simulink library "Contact_Forces_Lib"  (R2016a)
settings: Solver=ode45  StartTime=0.0  StopTime=10.0  RelTol=1e-3
undefined symbols (not defined in the file or in its folder): Extr_Data_Ring, radius_tube, X, Y, Z
undefined symbols (not defined in the file): b_contact, custom_param_1, custom_param_2, k_contact, l_cone, length_cylinder, length_tube, mu_kinetic, mu_static, pen_exponent, pen_full_damp_F, rad_s_cone, radius_cylinder, v_thr
libraries: nesl_utility x200, sm_lib x115, Contact_Forces_Lib x72, simulink x20, fl_lib x1
(part 10 of 12)

== system Contact_Forces_Lib/2D/Circle to Finite Line Force Enabled/Forces/Resolve Forces/Friction ==
  Unit Vector : Inport
  Fn : Inport  Port=2
  X Sep : Inport  Port=3
  vLin : Inport  Port=4
  wz : Inport  Port=5
  Components : Gain  Gain=[1 -1]
  Demux : Demux  Outputs=2
  Friction Law : Contact_Forces_Lib/Friction Law  OverrideUsingVariant=None
  Line Ref h : Gain  Gain=line_depth
  Product1 : Product
  Product2 : Product
  Product3 : Product
  Radius : Gain  Gain=-circle_rad
  Sign : Signum
  Sum : Sum  Inputs=-+
  VCirPt : Subsystem
  FxCir : Outport
  FyCir : Outport  Port=2
  FyLin : Outport  Port=3
  TzLin : Outport  Port=4
  TzCir : Outport  Port=5
  Ff : Outport  Port=6
  wires:
  Product3/1 -> Product2/1
  Components/1 -> Product3/1
  Product1/1 -> FyLin/1
  Friction Law/1 -> Line Ref h/1, Product2/2, Ff/1, Radius/1, Product1/1  "Ff"
  Demux/1 -> FyCir/1  "FyCir"
  vLin/1 -> Sum/1
  VCirPt/1(vCir) -> Sum/2
  Demux/2 -> FxCir/1  "FxCir"
  wz/1 -> VCirPt/1(wz)
  Unit Vector/1 -> Components/1
  Sum/1 -> Friction Law/2
  Fn/1 -> Friction Law/1
  Line Ref h/1 -> TzLin/1
  Radius/1 -> TzCir/1
  Product2/1 -> Demux/1
  X Sep/1 -> Sign/1, VCirPt/2(X sep)
  Sign/1 -> Product1/2, Product3/2

== system Contact_Forces_Lib/2D/Circle to Ring Force/Forces/Ff/Calculate vRel at CP  ==
  InOut : Inport
  rad : Inport  Port=2
  Pen : Inport  Port=3
  vazm : Inport  Port=4
  wzf : Inport  Port=5
  Follower Radius : Constant  Value=radius_circle
  Midpt Pen : Gain  Gain=0.5
  Product1 : Product
  Product2 : Product
  Product3 : Product
  Sum{,1..2,4} (4 alike) : Sum  Inputs=+-
  vRelCP : Outport
  rCirFtoCP : Outport  Port=2
  rRinBtoCP : Outport  Port=3
  wires:
  InOut/1 -> Product1/2  "InOut"
  Sum2/1 -> vRelCP/1
  Pen/1 -> Midpt Pen/1
  Sum/1 -> rRinBtoCP/1, Product2/2  "rRinBtoCP"
  rad/1 -> Sum/1
  Product2/1 -> Sum2/1  "vRelTra"
  Product3/1 -> Sum2/2  "vRelRot"
  Follower Radius/1 -> Sum1/1
  wzf/1 -> Sum4/1
  vazm/1 -> Product2/1, Sum4/2
  Midpt Pen/1 -> Sum1/2
  Sum4/1 -> Product3/1
  Product1/1 -> Sum/2, Product3/2  "rCirFtoCP sign"
  Sum1/1 -> rCirFtoCP/1, Product1/1  "rCirFtoCP"

== system Contact_Forces_Lib/2D/Circle to Ring Force/Forces/Ff/Resolve Ff ==
  note: Resolve Friction Force in
      | Circle B reference frame
      | Sign of Fn indicates
      | inside or outside ring.
  note: Resolve Friction Force in
      | Circle F reference frame
  Fn : Inport
  Ff : Inport  Port=2
  R : Inport  Port=3
  azm : Inport  Port=4
  rCirFtoCP : Inport  Port=5
  rRinBtoCP : Inport  Port=6
  Ff in CirB : Subsystem
  Ff in CirF : Subsystem
  Product : Product
  Sign : Signum  ZeroCross=off
  Tz : Subsystem
  FxCirF : Outport
  FyCirF : Outport  Port=2
  TzCirF : Outport  Port=3
  FxRinB : Outport  Port=4
  FyRinB : Outport  Port=5
  TzRinB : Outport  Port=6
  wires:
  Product/1 -> Ff in CirB/1(Ff)
  Sign/1 -> Product/2
  Fn/1 -> Sign/1
  Ff in CirF/1(FyCirF) -> FyCirF/1
  Ff in CirB/1(FxRinB) -> FxRinB/1, Ff in CirF/2(FxRinB)
  Ff in CirB/2(FyRinB) -> FyRinB/1, Ff in CirF/3(FyRinB)
  Ff in CirF/2(FxCirF) -> FxCirF/1
  Ff/1 -> Product/1, Tz/3(Ff)
  Tz/1(TzRinB) -> TzRinB/1
  Tz/2(TzCirF) -> TzCirF/1
  azm/1 -> Ff in CirB/2(azm)
  R/1 -> Ff in CirF/1(R)
  rCirFtoCP/1 -> Tz/1(rCirFtoCP)
  rRinBtoCP/1 -> Tz/2(rRinBtoCP)

== system Contact_Forces_Lib/2D/Circle to Ring Force/Forces/Fn/Fn in CirB ==
  Fn : Inport
  azm : Inport  Port=2
  Divide1 : Product  Inputs=**
  Divide2 : Product  Inputs=**
  Gain2 : Gain  Gain=-1
  cos : Trigonometry  Operator=cos
  deg2rad : Gain  Gain=pi/180
  sin : Trigonometry
  FxCirB : Outport
  FyCirB : Outport  Port=2
  wires:
  Gain2/1 -> Divide1/1, Divide2/1
  deg2rad/1 -> cos/1, sin/1
  sin/1 -> Divide2/2
  cos/1 -> Divide1/2
  Divide1/1 -> FxCirB/1
  Divide2/1 -> FyCirB/1
  Fn/1 -> Gain2/1
  azm/1 -> deg2rad/1

== system Contact_Forces_Lib/2D/Circle to Ring Force/Forces/Fn/Fn in CirF ==
  R : Inport
  FxCirB : Inport  Port=2
  FyCirB : Inport  Port=3
  Demux : Demux  Outputs=2
  Divide3 : Product  Inputs=**  Multiplication=Matrix(*)
  Gain : Gain  Gain=-1
  Mux1 : Mux  Inputs=2
  FyCirF : Outport
  FxCirF : Outport  Port=2
  wires:
  Demux/2 -> FxCirF/1
  Demux/1 -> FyCirF/1
  Gain/1 -> Demux/1
  Mux1/1 -> Divide3/2
  Divide3/1 -> Gain/1
  R/1 -> Divide3/1
  FyCirB/1 -> Mux1/1
  FxCirB/1 -> Mux1/2

== system Contact_Forces_Lib/2D/Composite Forces/Box to Belt Force/Belt Ends/Sensing C5 ==
  S : Inport
  Bus Selector : BusSelector  OutputSignals=Normal Force
  Fn : Outport
  wires:
  S/1 -> Bus Selector/1
  Bus Selector/1 -> Fn/1  "<Normal Force>"

== system Contact_Forces_Lib/2D/Composite Forces/Box to Belt Force/Belt Ends/Sensing C6 ==
  S : Inport
  Bus Selector : BusSelector  OutputSignals=Normal Force
  Fn : Outport
  wires:
  Bus Selector/1 -> Fn/1  "<Normal Force>"
  S/1 -> Bus Selector/1

== system Contact_Forces_Lib/2D/Composite Forces/Box to Belt Force/Belt Ends/Sensing C7 ==
  S : Inport
  Bus Selector : BusSelector  OutputSignals=Normal Force
  Fn : Outport
  wires:
  Bus Selector/1 -> Fn/1  "<Normal Force>"
  S/1 -> Bus Selector/1

== system Contact_Forces_Lib/2D/Composite Forces/Box to Belt Force/Belt Ends/Sensing C8 ==
  S : Inport
  Bus Selector : BusSelector  OutputSignals=Normal Force
  Fn : Outport
  wires:
  S/1 -> Bus Selector/1
  Bus Selector/1 -> Fn/1  "<Normal Force>"

== system Contact_Forces_Lib/2D/Composite Forces/Box to Belt Force/Belt Faces/Sensing C1 ==
  S : Inport
  Bus Selector : BusSelector  OutputSignals=Normal Force
  Fn : Outport
  wires:
  Bus Selector/1 -> Fn/1  "<Normal Force>"
  S/1 -> Bus Selector/1

== system Contact_Forces_Lib/2D/Composite Forces/Box to Belt Force/Belt Faces/Sensing C2 ==
  S : Inport
  Bus Selector : BusSelector  OutputSignals=Normal Force
  Fn : Outport
  wires:
  S/1 -> Bus Selector/1
  Bus Selector/1 -> Fn/1  "<Normal Force>"

== system Contact_Forces_Lib/2D/Composite Forces/Box to Belt Force/Belt Faces/Sensing C3 ==
  S : Inport
  Bus Selector : BusSelector  OutputSignals=Normal Force
  Fn : Outport
  wires:
  S/1 -> Bus Selector/1
  Bus Selector/1 -> Fn/1  "<Normal Force>"

== system Contact_Forces_Lib/2D/Composite Forces/Box to Belt Force/Belt Faces/Sensing C4 ==
  S : Inport
  Bus Selector : BusSelector  OutputSignals=Normal Force
  Fn : Outport
  wires:
  Bus Selector/1 -> Fn/1  "<Normal Force>"
  S/1 -> Bus Selector/1

== system Contact_Forces_Lib/2D/Composite Forces/Box to Box Force/BoxB Corners/Forces ==
  1AC : Inport
  1BD : Inport  Port=2
  2AC : Inport  Port=3
  2BD : Inport  Port=4
  3AC : Inport  Port=5
  3BD : Inport  Port=6
  4AC : Inport  Port=7
  4BD : Inport  Port=8
  Bus Creator : BusCreator  Inputs=8
  Bus Selector{1..8} (8 alike) : BusSelector  OutputSignals=FLin.Fx  OutputAsBus=on
  tag scope: FrcBC=scoped
  wires:
  Bus Creator/1 -> [FrcBC]
  Bus Selector7/1 -> Bus Creator/8  "BC4BD"
  4BD/1 -> Bus Selector7/1
  Bus Selector8/1 -> Bus Creator/7  "BC4AC"
  4AC/1 -> Bus Selector8/1
  Bus Selector5/1 -> Bus Creator/6  "BC3BD"
  3BD/1 -> Bus Selector5/1
  Bus Selector6/1 -> Bus Creator/5  "BC3AC"
  3AC/1 -> Bus Selector6/1
  Bus Selector3/1 -> Bus Creator/4  "BC2BD"
  2BD/1 -> Bus Selector3/1
  Bus Selector4/1 -> Bus Creator/3  "BC2AC"
  2AC/1 -> Bus Selector4/1
  Bus Selector1/1 -> Bus Creator/2  "BC1BD"
  1BD/1 -> Bus Selector1/1
  Bus Selector2/1 -> Bus Creator/1  "BC1AC"
  1AC/1 -> Bus Selector2/1

== system Contact_Forces_Lib/2D/Composite Forces/Box to Box Force/BoxF Corners/Forces ==
  1AC : Inport
  1BD : Inport  Port=2
  2AC : Inport  Port=3
  2BD : Inport  Port=4
  3AC : Inport  Port=5
  3BD : Inport  Port=6
  4AC : Inport  Port=7
  4BD : Inport  Port=8
  Bus Creator : BusCreator  Inputs=8
  Bus Selector{1..8} (8 alike) : BusSelector  OutputSignals=FLin.Fx  OutputAsBus=on
  tag scope: FrcFC=scoped
  wires:
  Bus Creator/1 -> [FrcFC]
  Bus Selector7/1 -> Bus Creator/8  "FC4BD"
  4BD/1 -> Bus Selector7/1
  Bus Selector8/1 -> Bus Creator/7  "FC4AC"
  4AC/1 -> Bus Selector8/1
  Bus Selector5/1 -> Bus Creator/6  "FC3BD"
  3BD/1 -> Bus Selector5/1
  Bus Selector6/1 -> Bus Creator/5  "FC3AC"
  3AC/1 -> Bus Selector6/1
  Bus Selector3/1 -> Bus Creator/4  "FC2BD"
  2BD/1 -> Bus Selector3/1
  Bus Selector4/1 -> Bus Creator/3  "FC2AC"
  2AC/1 -> Bus Selector4/1
  Bus Selector1/1 -> Bus Creator/2  "FC1BD"
  1BD/1 -> Bus Selector1/1
  Bus Selector2/1 -> Bus Creator/1  "FC1AC"
  1AC/1 -> Bus Selector2/1

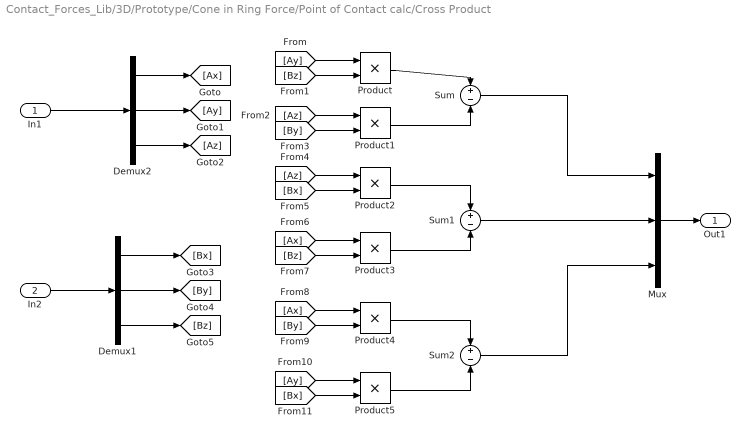
== system Contact_Forces_Lib/3D/Prototype/Cone in Ring Force/Point of Contact calc/Cross Product ==
  In1 : Inport
  In2 : Inport  Port=2
  Demux1 : Demux  Outputs=3
  Demux2 : Demux  Outputs=3
  Mux : Mux  Inputs=3
  Product{,1..5} (6 alike) : Product
  Sum : Sum  Inputs=+|-
  Sum1 : Sum  Inputs=+|-
  Sum2 : Sum  Inputs=+|-
  Out1 : Outport
  wires:
  [Bx] -> Product5/2
  [Ay] -> Product5/1
  [By] -> Product4/2
  [Ax] -> Product4/1
  [Bz] -> Product3/2
  [Ax] -> Product3/1
  [Bx] -> Product2/2
  [Az] -> Product2/1
  [By] -> Product1/2
  [Az] -> Product1/1
  [Bz] -> Product/2
  [Ay] -> Product/1
  Demux1/3 -> [Bz]
  Demux1/2 -> [By]
  Demux1/1 -> [Bx]
  Demux2/3 -> [Az]
  Demux2/2 -> [Ay]
  Demux2/1 -> [Ax]
  In1/1 -> Demux2/1
  Sum2/1 -> Mux/3
  Sum/1 -> Mux/1
  Sum1/1 -> Mux/2
  Product5/1 -> Sum2/2
  Product4/1 -> Sum2/1
  Product3/1 -> Sum1/2
  Product2/1 -> Sum1/1
  Product/1 -> Sum/1
  Product1/1 -> Sum/2
  Mux/1 -> Out1/1
  In2/1 -> Demux1/1

== system Contact_Forces_Lib/3D/Prototype/Cone in Ring Force/Point of Contact calc/Force Calc ==
  x : Inport
  y : Inport  Port=2
  r : Inport  Port=3
  z : Inport  Port=4
  th : Inport  Port=5
  Computing Force from nonzero penetration points : Subsystem  Commented=on
  Constant2 : Constant  Value=r_tube
  Dead Zone : DeadZone  LowerValue=-inf  UpperValue=0  ZeroCross=off  SaturateOnIntegerOverflow=on
  MAX_ML : Subsystem  Commented=on
  MAX_SL : Subsystem
  Math Function : Math  Operator=square  SaturateOnIntegerOverflow=on
  Math Function1 : Math  Operator=square  SaturateOnIntegerOverflow=on
  Reciprocal Sqrt : Sqrt  SaturateOnIntegerOverflow=on
  Sum : Sum  Inputs=|++
  Sum1 : Sum  Inputs=|+-
  Fx : Outport
  Fy : Outport  Port=2
  Fz : Outport  Port=3
  pc : Outport  Port=4
  wires:
  x/1 -> MAX_SL/2(X), Math Function/1
  Sum/1 -> Reciprocal Sqrt/1
  Reciprocal Sqrt/1 -> Sum1/1
  Constant2/1 -> Sum1/2
  Sum1/1 -> Dead Zone/1
  Math Function1/1 -> Sum/1
  Math Function/1 -> Sum/2
  y/1 -> Math Function1/1, MAX_SL/1(Y)
  MAX_SL/1(Fx) -> Fx/1
  MAX_SL/2(Fy) -> Fy/1
  Dead Zone/1 -> MAX_SL/3(Pen)
  MAX_SL/3(Fz) -> Fz/1
  MAX_SL/4(pc) -> pc/1
  r/1 -> MAX_SL/4(r)
  th/1 -> MAX_SL/5(th)
  z/1 -> MAX_SL/6(z)

== system Contact_Forces_Lib/3D/Prototype/Cone in Ring Force/Point of Contact calc/r calc ==
  note: r(z) = (z+l_cyl/2)(rl-rs)/lc +rl
  z : Inport
  Constant4 : Constant  Value=(rl + (l_cyl*(rl - rs))/(2*lc))
  Gain1 : Gain  Gain=(rl - rs)/lc
  Sum1 : Sum  Inputs=|++
  r : Outport
  wires:
  Constant4/1 -> Sum1/2
  Gain1/1 -> Sum1/1
  z/1 -> Gain1/1
  Sum1/1 -> r/1

== system Contact_Forces_Lib/3D/Prototype/Cone in Ring Force/Point of Contact calc/x calc ==
  r11 : Inport
  r12 : Inport  Port=2
  r13 : Inport  Port=3
  xc : Inport  Port=4
  th : Inport  Port=5
  z : Inport  Port=6
  r : Inport  Port=7
  Product{,1..4} (5 alike) : Product
  Sum : Sum  Inputs=|++++
  Trigonometric Function : Trigonometry  Operator=cos
  Trigonometric Function1 : Trigonometry
  x : Outport
  wires:
  th/1 -> Trigonometric Function1/1, Trigonometric Function/1
  Sum/1 -> x/1
  Product/1 -> Product3/1
  Product4/1 -> Sum/3
  Trigonometric Function/1 -> Product/2
  Trigonometric Function1/1 -> Product1/2
  Product3/1 -> Sum/2
  Product1/1 -> Product4/2
  r11/1 -> Product/1
  r12/1 -> Product1/1
  xc/1 -> Sum/1
  r13/1 -> Product2/1
  z/1 -> Product2/2
  Product2/1 -> Sum/4
  r/1 -> Product3/2, Product4/1

== system Contact_Forces_Lib/3D/Prototype/Cone in Ring Force/Point of Contact calc/y calc ==
  r21 : Inport
  r22 : Inport  Port=2
  r23 : Inport  Port=3
  yc : Inport  Port=4
  th : Inport  Port=5
  z : Inport  Port=6
  r : Inport  Port=7
  Product{,1..4} (5 alike) : Product
  Sum : Sum  Inputs=|++++
  Trigonometric Function : Trigonometry  Operator=cos
  Trigonometric Function1 : Trigonometry
  y : Outport
  wires:
  Product2/1 -> Sum/4
  z/1 -> Product2/2
  r23/1 -> Product2/1
  yc/1 -> Sum/1
  r22/1 -> Product1/1
  r21/1 -> Product/1
  Product1/1 -> Product4/2
  Product3/1 -> Sum/2
  Trigonometric Function1/1 -> Product1/2
  Trigonometric Function/1 -> Product/2
  Product4/1 -> Sum/3
  Product/1 -> Product3/1
  Sum/1 -> y/1
  th/1 -> Trigonometric Function1/1, Trigonometric Function/1
  r/1 -> Product3/2, Product4/1

== system Contact_Forces_Lib/3D/Prototype/Cone in Ring Force/Point of Contact calc/z calc ==
  note: num = -(Zc - L/2 + r31*cos(th)*(rl + (Lcyl*(rl - rs))/(2*lc)) + r32*sin(th)*(rl + (Lcyl*(rl - rs))/(2*lc)))
      | den = (r33 + (r31*cos(th)*(rl - rs))/lc + (r32*sin(th)*(rl - rs))/lc)
  r31 : Inport
  r32 : Inport  Port=2
  r33 : Inport  Port=3
  zc : Inport  Port=4
  th : Inport  Port=5
  Constant : Constant  Value=(rl + (l_cyl*(rl - rs))/(2*lc))
  Constant1 : Constant  Value=l_tube/2
  Constant2 : Constant  Value=(rl - rs)/lc
  Divide : Product  Inputs=*/
  Gain : Gain  Gain=-1
  Product{,1..5} (6 alike) : Product
  Sum : Sum  Inputs=+-++
  Sum1 : Sum  Inputs=+++
  Trigonometric Function : Trigonometry  Operator=cos
  Trigonometric Function1 : Trigonometry
  z : Outport
  wires:
  Divide/1 -> z/1
  th/1 -> Trigonometric Function1/1, Trigonometric Function/1
  Trigonometric Function/1 -> Product/2
  r31/1 -> Product/1
  Trigonometric Function1/1 -> Product1/2
  r32/1 -> Product1/1
  zc/1 -> Sum/1
  Constant1/1 -> Sum/2
  Product2/1 -> Sum/3
  Product3/1 -> Sum/4
  Product/1 -> Product4/1, Product2/1
  Product1/1 -> Product3/1, Product5/1
  Constant/1 -> Product3/2, Product2/2
  Sum/1 -> Gain/1
  Product5/1 -> Sum1/3
  Product4/1 -> Sum1/2
  r33/1 -> Sum1/1
  Constant2/1 -> Product4/2, Product5/2
  Sum1/1 -> Divide/2
  Gain/1 -> Divide/1

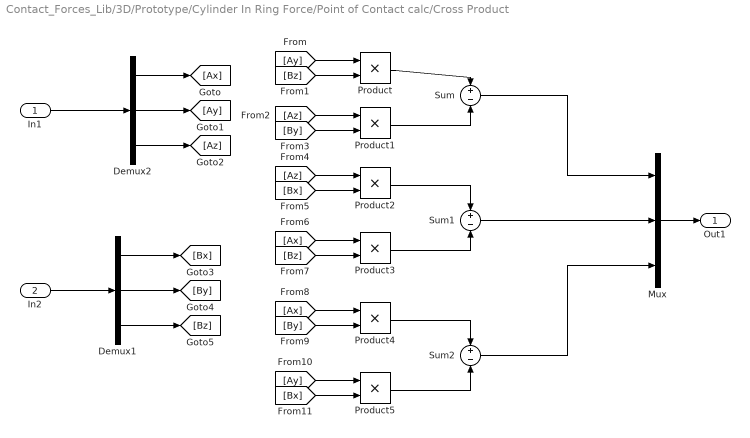
== system Contact_Forces_Lib/3D/Prototype/Cylinder In Ring Force/Point of Contact calc/Cross Product ==
  In1 : Inport
  In2 : Inport  Port=2
  Demux1 : Demux  Outputs=3
  Demux2 : Demux  Outputs=3
  Mux : Mux  Inputs=3
  Product{,1..5} (6 alike) : Product
  Sum : Sum  Inputs=+|-
  Sum1 : Sum  Inputs=+|-
  Sum2 : Sum  Inputs=+|-
  Out1 : Outport
  wires:
  [Bx] -> Product5/2
  [Ay] -> Product5/1
  [By] -> Product4/2
  [Ax] -> Product4/1
  [Bz] -> Product3/2
  [Ax] -> Product3/1
  [Bx] -> Product2/2
  [Az] -> Product2/1
  [By] -> Product1/2
  [Az] -> Product1/1
  [Bz] -> Product/2
  [Ay] -> Product/1
  Demux1/3 -> [Bz]
  Demux1/2 -> [By]
  Demux1/1 -> [Bx]
  Demux2/3 -> [Az]
  Demux2/2 -> [Ay]
  Demux2/1 -> [Ax]
  In1/1 -> Demux2/1
  Sum2/1 -> Mux/3
  Sum/1 -> Mux/1
  Sum1/1 -> Mux/2
  Product5/1 -> Sum2/2
  Product4/1 -> Sum2/1
  Product3/1 -> Sum1/2
  Product2/1 -> Sum1/1
  Product/1 -> Sum/1
  Product1/1 -> Sum/2
  Mux/1 -> Out1/1
  In2/1 -> Demux1/1

== system Contact_Forces_Lib/3D/Prototype/Cylinder In Ring Force/Point of Contact calc/Force Calc ==
  x : Inport
  y : Inport  Port=2
  v : Inport  Port=3
  z : Inport  Port=4
  th : Inport  Port=5
  Computing Force from nonzero penetration points : Subsystem  Commented=on
  Constant2 : Constant  Value=r_tube
  Dead Zone : DeadZone  LowerValue=-inf  UpperValue=0  ZeroCross=off  SaturateOnIntegerOverflow=on
  MAX_ML : Subsystem  Commented=on
  MAX_SL : Subsystem
  Math Function : Math  Operator=square  SaturateOnIntegerOverflow=on
  Math Function1 : Math  Operator=square  SaturateOnIntegerOverflow=on
  Reciprocal Sqrt : Sqrt  SaturateOnIntegerOverflow=on
  Sum : Sum  Inputs=|++
  Sum1 : Sum  Inputs=|+-
  Fx : Outport
  Fy : Outport  Port=2
  Fz : Outport  Port=3
  pc : Outport  Port=4
  maxpen : Outport  Port=5
  wires:
  y/1 -> MAX_SL/1(Y), Math Function1/1
  x/1 -> MAX_SL/2(X), Math Function/1
  Sum/1 -> Reciprocal Sqrt/1
  Reciprocal Sqrt/1 -> Sum1/1
  Constant2/1 -> Sum1/2
  Sum1/1 -> Dead Zone/1
  MAX_SL/1(Fx) -> Fx/1
  MAX_SL/2(Fy) -> Fy/1
  Dead Zone/1 -> MAX_SL/3(Pen)
  Math Function1/1 -> Sum/1
  Math Function/1 -> Sum/2
  v/1 -> MAX_SL/4(v)
  th/1 -> MAX_SL/5(th)
  z/1 -> MAX_SL/6(z)
  MAX_SL/4(pc) -> pc/1
  MAX_SL/3(Fz) -> Fz/1
  MAX_SL/5(maxpen) -> maxpen/1

== system Contact_Forces_Lib/3D/Prototype/Cylinder In Ring Force/Point of Contact calc/x calc ==
  note: Xb = r11*r*cos(th) + r12*r*sin(th) +r13*z + Xc;
  note: Find x coordinate in tube frame for cylinder point that is in the plane of the end of the tube
  r11 : Inport
  r12 : Inport  Port=2
  r13 : Inport  Port=3
  xc : Inport  Port=4
  th : Inport  Port=5
  z : Inport  Port=6
  Gain : Gain  Gain=r_cyl
  Gain1 : Gain  Gain=r_cyl
  Product : Product
  Product1 : Product
  Product2 : Product
  Sum : Sum  Inputs=|++++
  Trigonometric Function : Trigonometry  Operator=cos
  Trigonometric Function1 : Trigonometry
  x : Outport
  wires:
  th/1 -> Trigonometric Function/1, Trigonometric Function1/1
  Sum/1 -> x/1
  Product/1 -> Gain/1
  Gain1/1 -> Sum/3
  Trigonometric Function/1 -> Product/2
  Trigonometric Function1/1 -> Product1/2
  Gain/1 -> Sum/2
  Product1/1 -> Gain1/1
  r11/1 -> Product/1
  r12/1 -> Product1/1
  xc/1 -> Sum/1
  r13/1 -> Product2/1
  z/1 -> Product2/2
  Product2/1 -> Sum/4

== system Contact_Forces_Lib/3D/Prototype/Cylinder In Ring Force/Point of Contact calc/y calc ==
  note: Yb = r21*r*cos(th) + r22*r*sin(th) +r23*z + Yc;
  note: Find y coordinate in tube frame for cylinder point that is in the plane of the end of the tube
  r21 : Inport
  r22 : Inport  Port=2
  r23 : Inport  Port=3
  yc : Inport  Port=4
  th : Inport  Port=5
  z : Inport  Port=6
  Gain : Gain  Gain=r_cyl
  Gain1 : Gain  Gain=r_cyl
  Product : Product
  Product1 : Product
  Product2 : Product
  Sum : Sum  Inputs=|++++
  Trigonometric Function : Trigonometry  Operator=cos
  Trigonometric Function1 : Trigonometry
  y : Outport
  wires:
  Product2/1 -> Sum/4
  z/1 -> Product2/2
  r23/1 -> Product2/1
  yc/1 -> Sum/1
  r22/1 -> Product1/1
  r21/1 -> Product/1
  Product1/1 -> Gain1/1
  Gain/1 -> Sum/2
  Trigonometric Function1/1 -> Product1/2
  Trigonometric Function/1 -> Product/2
  Gain1/1 -> Sum/3
  Product/1 -> Gain/1
  Sum/1 -> y/1
  th/1 -> Trigonometric Function1/1, Trigonometric Function/1

== system Contact_Forces_Lib/3D/Prototype/Cylinder In Ring Force/Point of Contact calc/z calc ==
  note: Find z coordinate in cylinder frame for cylinder point that is in the plane of the end of the tube
  note: z = (L/2 - r31*r*cos(th) - r32*r*sin(th) - Zc)/r33;
  r31 : Inport
  r32 : Inport  Port=2
  r33 : Inport  Port=3
  zc : Inport  Port=4
  th : Inport  Port=5
  Constant : Constant  Value=l_tube/2
  Divide : Product  Inputs=*/
  Gain : Gain  Gain=r_cyl
  Gain1 : Gain  Gain=r_cyl
  Product : Product
  Product1 : Product
  Sum : Sum  Inputs=|---+
  Trigonometric Function : Trigonometry  Operator=cos
  Trigonometric Function1 : Trigonometry
  z : Outport
  wires:
  r32/1 -> Product1/1
  r31/1 -> Product/1
  Product1/1 -> Gain1/1
  Gain/1 -> Sum/2
  Trigonometric Function1/1 -> Product1/2
  Trigonometric Function/1 -> Product/2
  Gain1/1 -> Sum/3
  Product/1 -> Gain/1
  r33/1 -> Divide/2
  Constant/1 -> Sum/4
  Sum/1 -> Divide/1
  Divide/1 -> z/1
  zc/1 -> Sum/1
  th/1 -> Trigonometric Function1/1, Trigonometric Function/1

== system Contact_Forces_Lib/3D/Sphere in Sphere Force/Ff/Check w or v non zero/Else ==
  Action Port : ActionPort
  vabs_zero : Constant  Value=0  SampleTime=0
  vuvect_zero : Constant  Value=[0 0 0]  SampleTime=0
  vabs : Outport  InitialOutput=0
  vuvect : Outport  Port=2  InitialOutput=0
  wires:
  vabs_zero/1 -> vabs/1
  vuvect_zero/1 -> vuvect/1

== system Contact_Forces_Lib/3D/Sphere in Sphere Force/Ff/Check w or v non zero/mag v ==
  vect : Inport
  Add2 : Sum  Inputs=+++
  Demux : Demux  Outputs=3
  Math Function : Math  Operator=square  SaturateOnIntegerOverflow=on
  Math Function1 : Math  Operator=square  SaturateOnIntegerOverflow=on
  Math Function2 : Math  Operator=square  SaturateOnIntegerOverflow=on
  Sqrt : Sqrt  SaturateOnIntegerOverflow=on
  mag : Outport
  wires:
  Math Function2/1 -> Add2/3
  Demux/3 -> Math Function2/1
  Sqrt/1 -> mag/1
  Math Function1/1 -> Add2/2
  Math Function/1 -> Add2/1
  Add2/1 -> Sqrt/1
  vect/1 -> Demux/1
  Demux/1 -> Math Function/1
  Demux/2 -> Math Function1/1

== system Contact_Forces_Lib/3D/Sphere in Sphere Force/Ff/Check w or v non zero/mag w ==
  vect : Inport
  Add : Sum  Inputs=+++
  Demux : Demux  Outputs=3
  Math Function : Math  Operator=square  SaturateOnIntegerOverflow=on
  Math Function1 : Math  Operator=square  SaturateOnIntegerOverflow=on
  Math Function2 : Math  Operator=square  SaturateOnIntegerOverflow=on
  Sqrt : Sqrt  SaturateOnIntegerOverflow=on
  mag : Outport
  wires:
  Demux/2 -> Math Function1/1
  Demux/1 -> Math Function/1
  vect/1 -> Demux/1
  Add/1 -> Sqrt/1
  Math Function/1 -> Add/1
  Math Function1/1 -> Add/2
  Sqrt/1 -> mag/1
  Demux/3 -> Math Function2/1
  Math Function2/1 -> Add/3

== system Contact_Forces_Lib/3D/Sphere in Sphere Force/Ff/SlipVel/If Action Subsystem ==
  In1 : Inport
  In2 : Inport  Port=2
  Action Port : ActionPort
  Divide : Product  Inputs=/*
  Out1 : Outport
  wires:
  Divide/1 -> Out1/1
  In2/1 -> Divide/2
  In1/1 -> Divide/1

== system Contact_Forces_Lib/3D/Sphere in Sphere Force/Ff/SlipVel/mag ==
  vect : Inport
  Add2 : Sum  Inputs=+++
  Demux : Demux  Outputs=3
  Math Function : Math  Operator=square  SaturateOnIntegerOverflow=on
  Math Function1 : Math  Operator=square  SaturateOnIntegerOverflow=on
  Math Function2 : Math  Operator=square  SaturateOnIntegerOverflow=on
  Sqrt : Sqrt  SaturateOnIntegerOverflow=on
  mag : Outport
  wires:
  Math Function2/1 -> Add2/3
  Demux/3 -> Math Function2/1
  Sqrt/1 -> mag/1
  Math Function1/1 -> Add2/2
  Math Function/1 -> Add2/1
  Add2/1 -> Sqrt/1
  vect/1 -> Demux/1
  Demux/1 -> Math Function/1
  Demux/2 -> Math Function1/1

== system Contact_Forces_Lib/3D/Sphere to Cone Force/Forces/Ff/Relative vel at CP ==
  note: Calculate relative velocity at contact point between sphere and tube. Two components: about ring and along tube axis. Use magnitude to calculate friction force, atan2 retains relative magnitude and direction between the components.
  InOut : Inport
  rad : Inport  Port=2
  vrad : Inport  Port=3
  Pen : Inport  Port=4
  vazm : Inport  Port=5
  vazmx : Inport  Port=6
  vazmy : Inport  Port=7
  wzf : Inport  Port=8
  vzf : Inport  Port=9
  wxf : Inport  Port=10
  wyf : Inport  Port=11
  azm : Inport  Port=12
  Calculate vRelFace : Subsystem
  Calculate vRelRing : Subsystem
  Follower Radius : Constant  Value=radius_sphere
  Math Function : Math  Operator=square  SaturateOnIntegerOverflow=on
  Math Function1 : Math  Operator=square  SaturateOnIntegerOverflow=on
  Midpt Pen : Gain  Gain=0.5
  Product1 : Product
  Sqrt : Sqrt  SaturateOnIntegerOverflow=on
  Sum1 : Sum  Inputs=+-
  Sum3 : Sum  Inputs=|++
  Trigonometric Function : Trigonometry  Operator=atan2
  vRelAbs : Outport
  rSphtoCP : Outport  Port=2
  rConAxtoCP : Outport  Port=3
  alpha : Outport  Port=4
  wires:
  vrad/1 -> Calculate vRelFace/6(vrad)
  vazmy/1 -> Calculate vRelRing/6(vazmy)
  vazmx/1 -> Calculate vRelRing/5(vazmx)
  Product1/1 -> Calculate vRelRing/1(rSphtoCP sign), Calculate vRelFace/1(rSphtoCP sign)
  Sum1/1 -> Product1/1, rSphtoCP/1  "rSphtoCP"
  InOut/1 -> Product1/2  "InOut"
  Trigonometric Function/1 -> alpha/1  "alpha"
  Sqrt/1 -> vRelAbs/1
  Sum3/1 -> Sqrt/1
  Math Function/1 -> Sum3/1
  Math Function1/1 -> Sum3/2
  Follower Radius/1 -> Sum1/1
  Pen/1 -> Midpt Pen/1
  Midpt Pen/1 -> Sum1/2
  Calculate vRelFace/1(vRelFace) -> Math Function1/1, Trigonometric Function/1  "vRelFace"
  wxf/1 -> Calculate vRelFace/3(wxf), Calculate vRelRing/8(wxf)
  vzf/1 -> Calculate vRelFace/5(vzf)
  azm/1 -> Calculate vRelFace/2(azm), Calculate vRelRing/7(azm)
  wyf/1 -> Calculate vRelRing/9(wyf), Calculate vRelFace/4(wyf)
  Calculate vRelRing/2(vRelRing) -> Math Function/1, Trigonometric Function/2  "vRelRing"
  rad/1 -> Calculate vRelRing/2(rad)
  vazm/1 -> Calculate vRelRing/3(vazm)
  wzf/1 -> Calculate vRelRing/4(wzf)
  Calculate vRelRing/1(rConAxtoCP) -> rConAxtoCP/1

== system Contact_Forces_Lib/3D/Sphere to Cone Force/Forces/Ff/Resolve Ff ==
  note: Resolve Friction Force in
      | Sphere F reference frame
  note: Resolve Friction Force in
      | Cone B reference frame
  InOut : Inport
  Ff : Inport  Port=2
  R : Inport  Port=3
  z : Inport  Port=4
  rSphtoCP : Inport  Port=5
  rConAxtoCP : Inport  Port=6
  alpha : Inport  Port=7
  azm : Inport  Port=8
  Ff in ConB : Subsystem
  Ff in SphF : Subsystem
  FxSphF : Outport
  FySphF : Outport  Port=2
  FzSphF : Outport  Port=3
  TSphF : Outport  Port=4
  FxConB : Outport  Port=5
  FyConB : Outport  Port=6
  FzConB : Outport  Port=7
  TConB : Outport  Port=8
  wires:
  Ff in SphF/4(TSphF) -> TSphF/1
  Ff in ConB/4(TSphF_B) -> Ff in SphF/4(TSphF_B)
  Ff in ConB/5(TConB) -> TConB/1
  alpha/1 -> Ff in ConB/4(alpha)
  Ff in ConB/3(FzConB) -> FzConB/1, Ff in SphF/3(FzConB)
  Ff in SphF/3(FzSphF) -> FzSphF/1
  R/1 -> Ff in SphF/5(R)
  azm/1 -> Ff in ConB/3(azm)
  Ff in SphF/2(FxSphF) -> FxSphF/1
  Ff in ConB/2(FyConB) -> Ff in SphF/2(FyConB), FyConB/1
  Ff in ConB/1(FxConB) -> FxConB/1, Ff in SphF/1(FxConB)
  Ff in SphF/1(FySphF) -> FySphF/1
  Ff/1 -> Ff in ConB/2(Ff)
  rConAxtoCP/1 -> Ff in ConB/6(rConAxtoCP)
  rSphtoCP/1 -> Ff in ConB/5(rSphtoCP)
  z/1 -> Ff in ConB/7(z)
  InOut/1 -> Ff in ConB/1(InOut)

== system Contact_Forces_Lib/3D/Sphere to Cone Force/Forces/Fn/Equiv Torques ==
  azm : Inport
  FxConB : Inport  Port=2
  FyConB : Inport  Port=3
  FzConB : Inport  Port=4
  rad : Inport  Port=5
  z : Inport  Port=6
  Constant : Constant  Value=radius_sphere*sinConeTh
  Constant1 : Constant  Value=radius_sphere*cosConeTh
  Product : Product  Inputs=3
  Product1 : Product
  Product2 : Product  Inputs=3
  Product3 : Product
  Sum : Sum
  Sum1 : Sum  Inputs=+-
  Sum2 : Sum
  Sum3 : Sum  Inputs=+-
  sin : Trigonometry
  sin1 : Trigonometry  Operator=cos
  TxConB : Outport
  TyConB : Outport  Port=2
  wires:
  sin1/1 -> Product2/2
  sin/1 -> Product/2
  Sum/1 -> Product/3, Product2/3
  Sum3/1 -> TyConB/1
  Sum1/1 -> TxConB/1
  rad/1 -> Sum/1
  Product3/1 -> Sum3/1
  Product/1 -> Sum1/1
  Constant1/1 -> Sum2/2
  Sum2/1 -> Product3/2, Product1/2
  Constant/1 -> Sum/2
  z/1 -> Sum2/1
  Product1/1 -> Sum1/2
  Product2/1 -> Sum3/2
  azm/1 -> sin/1, sin1/1
  FxConB/1 -> Product3/1
  FzConB/1 -> Product/1, Product2/1
  FyConB/1 -> Product1/1

== system Contact_Forces_Lib/3D/Sphere to Cone Force/Forces/Fn/Fn in SphF ==
  R : Inport
  FxConB : Inport  Port=2
  FyConB : Inport  Port=3
  FzConB : Inport  Port=4
  Demux : Demux  Outputs=3
  Divide3 : Product  Inputs=/*  Multiplication=Matrix(*)
  Gain : Gain  Gain=-1
  Mux1 : Mux  Inputs=3
  FySphF : Outport
  FxSphF : Outport  Port=2
  FzSphF : Outport  Port=3
  wires:
  FzConB/1 -> Mux1/3
  Gain/1 -> Demux/1
  R/1 -> Divide3/1
  Demux/1 -> FxSphF/1
  Demux/2 -> FySphF/1
  Demux/3 -> FzSphF/1
  FxConB/1 -> Mux1/1
  FyConB/1 -> Mux1/2
  Mux1/1 -> Divide3/2
  Divide3/1 -> Gain/1

== system Contact_Forces_Lib/3D/Sphere to Cone Force/Forces/Fn/Fn in TubB ==
  Fn : Inport
  azm : Inport  Port=2
  Divide1 : Product  Inputs=**
  Divide2 : Product  Inputs=**
  Gain : Gain  Gain=sinConeTh
  Gain1 : Gain  Gain=sinConeTh
  cos : Trigonometry  Operator=cos
  sin : Trigonometry
  FxConB : Outport
  FyConB : Outport  Port=2
  FzConB : Outport  Port=3
  wires:
  Gain1/1 -> FzConB/1
  Gain/1 -> Divide1/1, Divide2/1
  Fn/1 -> Gain/1, Gain1/1
  azm/1 -> cos/1, sin/1
  sin/1 -> Divide2/2
  cos/1 -> Divide1/2
  Divide1/1 -> FxConB/1
  Divide2/1 -> FyConB/1

== system Contact_Forces_Lib/3D/Sphere to Cone Force/Sensing/rad_azm_cal/rad_0 ==
  Action Port : ActionPort
  Zeros : Constant  Value=[0 0 0 0]  SampleTime=0
  F : Outport  InitialOutput=[0]
  wires:
  Zeros/1 -> F/1

== system Contact_Forces_Lib/3D/Sphere to Cone Force/Sensing/rad_azm_cal/rad_azm_cal ==
  note: vazm = (x*vy - y*vx)/(x^2+y^2)
  note: vrad = (x*vx + y*vy)/z
  note: azm = atan2(y, x)
  note: rad = sqrt(x^2+y^2)
  x : Inport
  y : Inport  Port=2
  vx : Inport  Port=3
  vy : Inport  Port=4
  Action Port : ActionPort
  Add : Sum
  Add1 : Sum  Inputs=+-
  Divide : Product  Inputs=*/
  Divide1 : Product  Inputs=*/
  Math Function : Math  Operator=square  SaturateOnIntegerOverflow=on
  Math Function1 : Math  Operator=square  SaturateOnIntegerOverflow=on
  Mux : Mux
  Product{,1..3} (4 alike) : Product
  Sqrt : Sqrt  SaturateOnIntegerOverflow=on
  Sum : Sum
  Trigonometric Function : Trigonometry  Operator=atan2
  F : Outport
  wires:
  Math Function1/1 -> Sum/2
  Math Function/1 -> Sum/1
  Sum/1 -> Divide1/2, Sqrt/1
  Trigonometric Function/1 -> Mux/2  "azm"
  x/1 -> Trigonometric Function/2, Product/1, Product2/1, Math Function/1
  y/1 -> Trigonometric Function/1, Product1/1, Product3/1, Math Function1/1
  vx/1 -> Product3/2, Product/2
  vy/1 -> Product2/2, Product1/2
  Product/1 -> Add/1
  Product1/1 -> Add/2
  Add/1 -> Divide/1
  Sqrt/1 -> Mux/1, Divide/2  "rad"
  Divide/1 -> Mux/3  "vrad"
  Product2/1 -> Add1/1
  Product3/1 -> Add1/2
  Add1/1 -> Divide1/1
  Divide1/1 -> Mux/4  "vazm"
  Mux/1 -> F/1

== system Contact_Forces_Lib/3D/Sphere to Cone Force/Sensing/rad_azm_cal/vazmx_0 ==
  Action Port : ActionPort
  Zeros : Constant  Value=0  SampleTime=0
  F : Outport  InitialOutput=[0]
  wires:
  Zeros/1 -> F/1

== system Contact_Forces_Lib/3D/Sphere to Cone Force/Sensing/rad_azm_cal/vazmx_cal ==
  note: vazmx = (y*vz - z*vy)/(y^2+z^2)
  y : Inport
  z : Inport  Port=2
  vy : Inport  Port=3
  vz : Inport  Port=4
  Action Port : ActionPort
  Add2 : Sum  Inputs=+-
  Divide2 : Product  Inputs=*/
  Math Function1 : Math  Operator=square  SaturateOnIntegerOverflow=on
  Math Function2 : Math  Operator=square  SaturateOnIntegerOverflow=on
  Product4 : Product
  Product5 : Product
  Sum1 : Sum
  vazmx : Outport
  wires:
  Product4/1 -> Add2/1
  Product5/1 -> Add2/2
  Add2/1 -> Divide2/1
  vy/1 -> Product5/2
  y/1 -> Math Function1/1, Product4/1
  Math Function1/1 -> Sum1/1
  z/1 -> Product5/1, Math Function2/1
  Math Function2/1 -> Sum1/2
  Sum1/1 -> Divide2/2
  vz/1 -> Product4/2
  Divide2/1 -> vazmx/1  "vazmx"

== system Contact_Forces_Lib/3D/Sphere to Cone Force/Sensing/rad_azm_cal/vazmy_0 ==
  Action Port : ActionPort
  Zeros : Constant  Value=0  SampleTime=0
  F : Outport  InitialOutput=[0]
  wires:
  Zeros/1 -> F/1

== system Contact_Forces_Lib/3D/Sphere to Cone Force/Sensing/rad_azm_cal/vazmy_cal ==
  note: vazmy = (z*vx - x*vz)/(z^2+x^2)
  x : Inport
  z : Inport  Port=2
  vx : Inport  Port=3
  vz : Inport  Port=4
  Action Port : ActionPort
  Add3 : Sum  Inputs=+-
  Divide3 : Product  Inputs=*/
  Math Function : Math  Operator=square  SaturateOnIntegerOverflow=on
  Math Function2 : Math  Operator=square  SaturateOnIntegerOverflow=on
  Product6 : Product
  Product7 : Product
  Sum2 : Sum
  vazmy : Outport
  wires:
  vx/1 -> Product6/2
  x/1 -> Math Function/1, Product7/1
  Math Function/1 -> Sum2/1
  Add3/1 -> Divide3/1
  Product7/1 -> Add3/2
  Product6/1 -> Add3/1
  z/1 -> Product6/1, Math Function2/1
  Math Function2/1 -> Sum2/2
  Sum2/1 -> Divide3/2
  vz/1 -> Product7/2
  Divide3/1 -> vazmy/1  "vazmy"

== system Contact_Forces_Lib/3D/Sphere to Plane Force/Forces/Ff/SlipVel ==
  wx : Inport
  wy : Inport  Port=2
  vx : Inport  Port=3
  vy : Inport  Port=4
  Fx1 : Constant  Value=sphere_rad
  Math Function : Math  Operator=square  SaturateOnIntegerOverflow=on
  Math Function1 : Math  Operator=square  SaturateOnIntegerOverflow=on
  Product3 : Product
  Product4 : Product
  Sqrt : Sqrt  SaturateOnIntegerOverflow=on
  Sum1 : Sum  Inputs=|++
  Sum2 : Sum  Inputs=|-+
  Sum3 : Sum  Inputs=|++
  Trigonometric Function : Trigonometry  Operator=atan2
  vabs : Outport
  alpha : Outport  Port=2
  wires:
  Sum2/1 -> Math Function1/1, Trigonometric Function/2  "slipx"
  Sum1/1 -> Math Function/1, Trigonometric Function/1  "slipy"
  Math Function1/1 -> Sum3/2
  Math Function/1 -> Sum3/1
  Sum3/1 -> Sqrt/1
  Sqrt/1 -> vabs/1
  Trigonometric Function/1 -> alpha/1
  Product4/1 -> Sum2/1
  vy/1 -> Sum1/2
  Fx1/1 -> Product4/1, Product3/2
  vx/1 -> Sum2/2
  wy/1 -> Product4/2
  Product3/1 -> Sum1/1
  wx/1 -> Product3/1

== system Contact_Forces_Lib/3D/Sphere to Plane Force Enabled/Forces/Ff/SlipVel ==
  wx : Inport
  wy : Inport  Port=2
  vx : Inport  Port=3
  vy : Inport  Port=4
  Fx1 : Constant  Value=sphere_rad
  Math Function : Math  Operator=square  SaturateOnIntegerOverflow=on
  Math Function1 : Math  Operator=square  SaturateOnIntegerOverflow=on
  Product3 : Product
  Product4 : Product
  Sqrt : Sqrt  SaturateOnIntegerOverflow=on
  Sum1 : Sum  Inputs=|++
  Sum2 : Sum  Inputs=|-+
  Sum3 : Sum  Inputs=|++
  Trigonometric Function : Trigonometry  Operator=atan2
  vabs : Outport
  alpha : Outport  Port=2
  wires:
  wx/1 -> Product3/1
  Product3/1 -> Sum1/1
  wy/1 -> Product4/2
  vx/1 -> Sum2/2
  Fx1/1 -> Product3/2, Product4/1
  vy/1 -> Sum1/2
  Product4/1 -> Sum2/1
  Trigonometric Function/1 -> alpha/1
  Sqrt/1 -> vabs/1
  Sum3/1 -> Sqrt/1
  Math Function/1 -> Sum3/1
  Math Function1/1 -> Sum3/2
  Sum1/1 -> Trigonometric Function/1, Math Function/1  "slipy"
  Sum2/1 -> Trigonometric Function/2, Math Function1/1  "slipx"

== system Contact_Forces_Lib/3D/Sphere to Sphere Force/Ff/Check w or v non zero/Else ==
  Action Port : ActionPort
  Constant : Constant  Value=0  SampleTime=0
  Constant1 : Constant  Value=[0 0 0]  SampleTime=0
  vabs : Outport  InitialOutput=0
  vuvect : Outport  Port=2  InitialOutput=0
  wires:
  Constant1/1 -> vuvect/1
  Constant/1 -> vabs/1

== system Contact_Forces_Lib/3D/Sphere to Sphere Force/Ff/Check w or v non zero/mag v ==
  vect : Inport
  Add2 : Sum  Inputs=+++
  Demux : Demux  Outputs=3
  Math Function : Math  Operator=square  SaturateOnIntegerOverflow=on
  Math Function1 : Math  Operator=square  SaturateOnIntegerOverflow=on
  Math Function2 : Math  Operator=square  SaturateOnIntegerOverflow=on
  Sqrt : Sqrt  SaturateOnIntegerOverflow=on
  mag : Outport
  wires:
  Demux/2 -> Math Function1/1
  Demux/1 -> Math Function/1
  vect/1 -> Demux/1
  Add2/1 -> Sqrt/1
  Math Function/1 -> Add2/1
  Math Function1/1 -> Add2/2
  Sqrt/1 -> mag/1
  Demux/3 -> Math Function2/1
  Math Function2/1 -> Add2/3

== system Contact_Forces_Lib/3D/Sphere to Sphere Force/Ff/Check w or v non zero/mag w ==
  vect : Inport
  Add : Sum  Inputs=+++
  Demux : Demux  Outputs=3
  Math Function : Math  Operator=square  SaturateOnIntegerOverflow=on
  Math Function1 : Math  Operator=square  SaturateOnIntegerOverflow=on
  Math Function2 : Math  Operator=square  SaturateOnIntegerOverflow=on
  Sqrt : Sqrt  SaturateOnIntegerOverflow=on
  mag : Outport
  wires:
  Math Function2/1 -> Add/3
  Demux/3 -> Math Function2/1
  Sqrt/1 -> mag/1
  Math Function1/1 -> Add/2
  Math Function/1 -> Add/1
  Add/1 -> Sqrt/1
  vect/1 -> Demux/1
  Demux/1 -> Math Function/1
  Demux/2 -> Math Function1/1

== system Contact_Forces_Lib/3D/Sphere to Sphere Force/Ff/SlipVel/If Action Subsystem ==
  In1 : Inport
  In2 : Inport  Port=2
  Action Port : ActionPort
  Divide : Product  Inputs=/*
  Out1 : Outport
  wires:
  In1/1 -> Divide/1
  In2/1 -> Divide/2
  Divide/1 -> Out1/1

== system Contact_Forces_Lib/3D/Sphere to Sphere Force/Ff/SlipVel/mag ==
  vect : Inport
  Add2 : Sum  Inputs=+++
  Demux : Demux  Outputs=3
  Math Function : Math  Operator=square  SaturateOnIntegerOverflow=on
  Math Function1 : Math  Operator=square  SaturateOnIntegerOverflow=on
  Math Function2 : Math  Operator=square  SaturateOnIntegerOverflow=on
  Sqrt : Sqrt  SaturateOnIntegerOverflow=on
  mag : Outport
  wires:
  Demux/2 -> Math Function1/1
  Demux/1 -> Math Function/1
  vect/1 -> Demux/1
  Add2/1 -> Sqrt/1
  Math Function/1 -> Add2/1
  Math Function1/1 -> Add2/2
  Sqrt/1 -> mag/1
  Demux/3 -> Math Function2/1
  Math Function2/1 -> Add2/3

== system Contact_Forces_Lib/3D/Sphere to Tube Force/Forces/Ff/Relative vel at CP ==
  note: Calculate relative velocity at contact point between sphere and tube. Two components: about ring and along tube axis. Use magnitude to calculate friction force, atan2 retains relative magnitude and direction between the components.
  Fn : Inport
  rad : Inport  Port=2
  Pen : Inport  Port=3
  vazm : Inport  Port=4
  wzf : Inport  Port=5
  vzf : Inport  Port=6
  wxf : Inport  Port=7
  wyf : Inport  Port=8
  azm : Inport  Port=9
  Calculate vRelAxis : Subsystem
  Calculate vRelRing : Subsystem
  Follower Radius : Constant  Value=radius_sphere
  Math Function : Math  Operator=square  SaturateOnIntegerOverflow=on
  Math Function1 : Math  Operator=square  SaturateOnIntegerOverflow=on
  Midpt Pen : Gain  Gain=0.5
  Product1 : Product
  Sign : Signum  ZeroCross=off
  Sqrt : Sqrt  SaturateOnIntegerOverflow=on
  Sum1 : Sum  Inputs=+-
  Sum3 : Sum  Inputs=|++
  Trigonometric Function : Trigonometry  Operator=atan2
  vRelAbs : Outport
  rSphtoCP : Outport  Port=2
  rCyltoCP : Outport  Port=3
  alpha : Outport  Port=4
  wires:
  Calculate vRelRing/1(rCyltoCP) -> rCyltoCP/1
  wzf/1 -> Calculate vRelRing/3(wzf)
  vazm/1 -> Calculate vRelRing/2(vazm)
  rad/1 -> Calculate vRelRing/1(rad)
  Calculate vRelRing/2(vRelRing) -> Math Function/1, Trigonometric Function/2  "vRelRing"
  wyf/1 -> Calculate vRelAxis/5(wyf)
  azm/1 -> Calculate vRelAxis/4(azm)
  vzf/1 -> Calculate vRelAxis/3(vzf)
  wxf/1 -> Calculate vRelAxis/2(wxf)
  Calculate vRelAxis/1(vRelAxis) -> Trigonometric Function/1, Math Function1/1  "vRelAxis"
  Midpt Pen/1 -> Sum1/2
  Fn/1 -> Sign/1
  Pen/1 -> Midpt Pen/1
  Follower Radius/1 -> Sum1/1
  Math Function1/1 -> Sum3/2
  Math Function/1 -> Sum3/1
  Sum3/1 -> Sqrt/1
  Sqrt/1 -> vRelAbs/1
  Trigonometric Function/1 -> alpha/1  "alpha"
  Sign/1 -> Product1/2  "InOut"
  Sum1/1 -> Product1/1, rSphtoCP/1  "rSphtoCP"
  Product1/1 -> Calculate vRelAxis/1(rSphtoCP sign), Calculate vRelRing/4(rSphtoCP sign)

== system Contact_Forces_Lib/3D/Sphere to Tube Force/Forces/Ff/Resolve Ff ==
  note: Resolve Friction Force in
      | Tube B reference frame
  note: Resolve Friction Force in
      | Sphere F reference frame
  InOut : Inport
  Ff : Inport  Port=2
  rSphtoCP : Inport  Port=3
  rCyltoCP : Inport  Port=4
  alpha : Inport  Port=5
  z : Inport  Port=6
  R : Inport  Port=7
  azm : Inport  Port=8
  Ff in SphF : Subsystem
  Ff in TubB : Subsystem
  FxSphF : Outport
  FySphF : Outport  Port=2
  FzSphF : Outport  Port=3
  TSphF : Outport  Port=4
  FxSphB : Outport  Port=5
  FyTubB : Outport  Port=6
  FzTubB : Outport  Port=7
  TTubB : Outport  Port=8
  wires:
  InOut/1 -> Ff in TubB/1(InOut)
  z/1 -> Ff in TubB/7(z)
  rSphtoCP/1 -> Ff in TubB/5(rSphtoCP)
  rCyltoCP/1 -> Ff in TubB/6(rCyltoCP)
  Ff/1 -> Ff in TubB/2(Ff)
  Ff in SphF/1(FySphF) -> FySphF/1
  Ff in TubB/1(FxTubB) -> Ff in SphF/1(FxTubB), FxSphB/1
  Ff in TubB/2(FyTubB) -> FyTubB/1, Ff in SphF/2(FyTubB)
  Ff in SphF/2(FxSphF) -> FxSphF/1
  azm/1 -> Ff in TubB/3(azm)
  R/1 -> Ff in SphF/5(R)
  Ff in SphF/3(FzSphF) -> FzSphF/1
  Ff in TubB/3(FzTubB) -> Ff in SphF/3(FzTubB), FzTubB/1
  alpha/1 -> Ff in TubB/4(alpha)
  Ff in TubB/5(TTubB) -> TTubB/1
  Ff in TubB/4(TSphF_B) -> Ff in SphF/4(TSphF_B)
  Ff in SphF/4(TSphF) -> TSphF/1

== system Contact_Forces_Lib/3D/Sphere to Tube Force/Forces/Fn/Fn in SphF ==
  R : Inport
  FxTubB : Inport  Port=2
  FyTubB : Inport  Port=3
  Constant : Constant  Value=0
  Demux : Demux  Outputs=3
  Divide3 : Product  Inputs=/*  Multiplication=Matrix(*)
  Gain : Gain  Gain=-1
  Mux1 : Mux  Inputs=3
  FySphF : Outport
  FxSphF : Outport  Port=2
  FzSphF : Outport  Port=3
  wires:
  Divide3/1 -> Gain/1
  Mux1/1 -> Divide3/2
  FyTubB/1 -> Mux1/2
  FxTubB/1 -> Mux1/1
  Demux/3 -> FzSphF/1
  Demux/2 -> FySphF/1
  Demux/1 -> FxSphF/1
  Constant/1 -> Mux1/3
  R/1 -> Divide3/1
  Gain/1 -> Demux/1

== system Contact_Forces_Lib/3D/Sphere to Tube Force/Forces/Fn/Fn in TubB ==
  Fn : Inport
  azm : Inport  Port=2
  Divide1 : Product  Inputs=**
  Divide2 : Product  Inputs=**
  cos : Trigonometry  Operator=cos
  sin : Trigonometry
  FxTubB : Outport
  FyTubB : Outport  Port=2
  wires:
  Divide2/1 -> FyTubB/1
  Divide1/1 -> FxTubB/1
  cos/1 -> Divide1/2
  sin/1 -> Divide2/2
  azm/1 -> sin/1, cos/1
  Fn/1 -> Divide2/1, Divide1/1

== system Contact_Forces_Lib/3D/Sphere to Tube Force/Sensing/rad_azm_cal/rad_0 ==
  Action Port : ActionPort
  Zeros : Constant  Value=[0 0 0 0]  SampleTime=0
  F : Outport  InitialOutput=[0]
  wires:
  Zeros/1 -> F/1

== system Contact_Forces_Lib/3D/Sphere to Tube Force/Sensing/rad_azm_cal/rad_azm_cal ==
  note: z = sqrt(x2+y2)
      | zdot = 1/z(x*xdot+y*ydot)
      | azm = atan(y/x)
      | azmdot = 1/z2(x*ydot-xdot*y)
  X : Inport
  Y : Inport  Port=2
  Xdot : Inport  Port=3
  Ydot : Inport  Port=4
  Action Port : ActionPort
  Add : Sum
  Add1 : Sum  Inputs=+-
  Divide : Product  Inputs=*/
  Divide1 : Product  Inputs=*/
  Math Function : Math  Operator=square  SaturateOnIntegerOverflow=on
  Math Function1 : Math  Operator=square  SaturateOnIntegerOverflow=on
  Mux : Mux
  Product{,1..3} (4 alike) : Product
  Sqrt : Sqrt  SaturateOnIntegerOverflow=on
  Sum : Sum  Inputs=|++
  Trigonometric Function : Trigonometry  Operator=atan2
  F : Outport
  wires:
  Mux/1 -> F/1
  Divide1/1 -> Mux/4
  Add1/1 -> Divide1/1
  Product3/1 -> Add1/2
  Product2/1 -> Add1/1
  Divide/1 -> Mux/3
  Sqrt/1 -> Divide/2, Mux/1
  Add/1 -> Divide/1
  Product1/1 -> Add/2
  Product/1 -> Add/1
  Ydot/1 -> Product1/2, Product2/2
  Xdot/1 -> Product/2, Product3/2
  Y/1 -> Math Function1/1, Product1/1, Product3/1, Trigonometric Function/1
  X/1 -> Math Function/1, Product/1, Product2/1, Trigonometric Function/2
  Trigonometric Function/1 -> Mux/2
  Sum/1 -> Sqrt/1, Divide1/2
  Math Function/1 -> Sum/1
  Math Function1/1 -> Sum/2

== system Contact_Forces_Lib/3D/Sphere to Tube Force Enabled/Forces/Ff/Relative vel at CP ==
  note: Calculate relative velocity at contact point between sphere and tube. Two components: about ring and along tube axis. Use magnitude to calculate friction force, atan2 retains relative magnitude and direction between the components.
  Fn : Inport
  rad : Inport  Port=2
  Pen : Inport  Port=3
  vazm : Inport  Port=4
  wzf : Inport  Port=5
  vzf : Inport  Port=6
  wxf : Inport  Port=7
  wyf : Inport  Port=8
  azm : Inport  Port=9
  Calculate vRelAxis : Subsystem
  Calculate vRelRing : Subsystem
  Follower Radius : Constant  Value=radius_sphere
  Math Function : Math  Operator=square  SaturateOnIntegerOverflow=on
  Math Function1 : Math  Operator=square  SaturateOnIntegerOverflow=on
  Midpt Pen : Gain  Gain=0.5
  Product1 : Product
  Sign : Signum  ZeroCross=off
  Sqrt : Sqrt  SaturateOnIntegerOverflow=on
  Sum1 : Sum  Inputs=+-
  Sum3 : Sum  Inputs=|++
  Trigonometric Function : Trigonometry  Operator=atan2
  vRelAbs : Outport
  rSphtoCP : Outport  Port=2
  rCyltoCP : Outport  Port=3
  alpha : Outport  Port=4
  wires:
  Calculate vRelRing/1(rCyltoCP) -> rCyltoCP/1
  wzf/1 -> Calculate vRelRing/3(wzf)
  vazm/1 -> Calculate vRelRing/2(vazm)
  rad/1 -> Calculate vRelRing/1(rad)
  Calculate vRelRing/2(vRelRing) -> Math Function/1, Trigonometric Function/2  "vRelRing"
  wyf/1 -> Calculate vRelAxis/5(wyf)
  azm/1 -> Calculate vRelAxis/4(azm)
  vzf/1 -> Calculate vRelAxis/3(vzf)
  wxf/1 -> Calculate vRelAxis/2(wxf)
  Calculate vRelAxis/1(vRelAxis) -> Trigonometric Function/1, Math Function1/1  "vRelAxis"
  Midpt Pen/1 -> Sum1/2
  Fn/1 -> Sign/1
  Pen/1 -> Midpt Pen/1
  Follower Radius/1 -> Sum1/1
  Math Function1/1 -> Sum3/2
  Math Function/1 -> Sum3/1
  Sum3/1 -> Sqrt/1
  Sqrt/1 -> vRelAbs/1
  Trigonometric Function/1 -> alpha/1  "alpha"
  Sign/1 -> Product1/2  "InOut"
  Sum1/1 -> Product1/1, rSphtoCP/1  "rSphtoCP"
  Product1/1 -> Calculate vRelAxis/1(rSphtoCP sign), Calculate vRelRing/4(rSphtoCP sign)

== system Contact_Forces_Lib/3D/Sphere to Tube Force Enabled/Forces/Ff/Resolve Ff ==
  note: Resolve Friction Force in
      | Tube B reference frame
  note: Resolve Friction Force in
      | Sphere F reference frame
  InOut : Inport
  Ff : Inport  Port=2
  rSphtoCP : Inport  Port=3
  rCyltoCP : Inport  Port=4
  alpha : Inport  Port=5
  z : Inport  Port=6
  R : Inport  Port=7
  azm : Inport  Port=8
  Ff in SphF : Subsystem
  Ff in TubB : Subsystem
  FxSphF : Outport
  FySphF : Outport  Port=2
  FzSphF : Outport  Port=3
  TSphF : Outport  Port=4
  FxSphB : Outport  Port=5
  FyTubB : Outport  Port=6
  FzTubB : Outport  Port=7
  TTubB : Outport  Port=8
  wires:
  InOut/1 -> Ff in TubB/1(InOut)
  z/1 -> Ff in TubB/7(z)
  rSphtoCP/1 -> Ff in TubB/5(rSphtoCP)
  rCyltoCP/1 -> Ff in TubB/6(rCyltoCP)
  Ff/1 -> Ff in TubB/2(Ff)
  Ff in SphF/1(FySphF) -> FySphF/1
  Ff in TubB/1(FxTubB) -> Ff in SphF/1(FxTubB), FxSphB/1
  Ff in TubB/2(FyTubB) -> FyTubB/1, Ff in SphF/2(FyTubB)
  Ff in SphF/2(FxSphF) -> FxSphF/1
  azm/1 -> Ff in TubB/3(azm)
  R/1 -> Ff in SphF/5(R)
  Ff in SphF/3(FzSphF) -> FzSphF/1
  Ff in TubB/3(FzTubB) -> Ff in SphF/3(FzTubB), FzTubB/1
  alpha/1 -> Ff in TubB/4(alpha)
  Ff in TubB/5(TTubB) -> TTubB/1
  Ff in TubB/4(TSphF_B) -> Ff in SphF/4(TSphF_B)
  Ff in SphF/4(TSphF) -> TSphF/1

== system Contact_Forces_Lib/3D/Sphere to Tube Force Enabled/Forces/Fn/Fn in SphF ==
  R : Inport
  FxTubB : Inport  Port=2
  FyTubB : Inport  Port=3
  Constant : Constant  Value=0
  Demux : Demux  Outputs=3
  Divide3 : Product  Inputs=/*  Multiplication=Matrix(*)
  Gain : Gain  Gain=-1
  Mux1 : Mux  Inputs=3
  FySphF : Outport
  FxSphF : Outport  Port=2
  FzSphF : Outport  Port=3
  wires:
  Divide3/1 -> Gain/1
  Mux1/1 -> Divide3/2
  FyTubB/1 -> Mux1/2
  FxTubB/1 -> Mux1/1
  Demux/3 -> FzSphF/1
  Demux/2 -> FySphF/1
  Demux/1 -> FxSphF/1
  Constant/1 -> Mux1/3
  R/1 -> Divide3/1
  Gain/1 -> Demux/1

== system Contact_Forces_Lib/3D/Sphere to Tube Force Enabled/Forces/Fn/Fn in TubB ==
  Fn : Inport
  azm : Inport  Port=2
  Divide1 : Product  Inputs=**
  Divide2 : Product  Inputs=**
  cos : Trigonometry  Operator=cos
  sin : Trigonometry
  FxTubB : Outport
  FyTubB : Outport  Port=2
  wires:
  Divide2/1 -> FyTubB/1
  Divide1/1 -> FxTubB/1
  cos/1 -> Divide1/2
  sin/1 -> Divide2/2
  azm/1 -> sin/1, cos/1
  Fn/1 -> Divide2/1, Divide1/1

== system Contact_Forces_Lib/3D/Sphere to Tube Force Enabled/Sensing/rad_azm_cal/rad_0 ==
  Action Port : ActionPort
  Zeros : Constant  Value=[0 0 0 0]  SampleTime=0
  F : Outport  InitialOutput=[0]
  wires:
  Zeros/1 -> F/1

== system Contact_Forces_Lib/3D/Sphere to Tube Force Enabled/Sensing/rad_azm_cal/rad_azm_cal ==
  note: z = sqrt(x2+y2)
      | zdot = 1/z(x*xdot+y*ydot)
      | azm = atan(y/x)
      | azmdot = 1/z2(x*ydot-xdot*y)
  X : Inport
  Y : Inport  Port=2
  Xdot : Inport  Port=3
  Ydot : Inport  Port=4
  Action Port : ActionPort
  Add : Sum
  Add1 : Sum  Inputs=+-
  Divide : Product  Inputs=*/
  Divide1 : Product  Inputs=*/
  Math Function : Math  Operator=square  SaturateOnIntegerOverflow=on
  Math Function1 : Math  Operator=square  SaturateOnIntegerOverflow=on
  Mux : Mux
  Product{,1..3} (4 alike) : Product
  Sqrt : Sqrt  SaturateOnIntegerOverflow=on
  Sum : Sum  Inputs=|++
  Trigonometric Function : Trigonometry  Operator=atan2
  F : Outport
  wires:
  Mux/1 -> F/1
  Divide1/1 -> Mux/4
  Add1/1 -> Divide1/1
  Product3/1 -> Add1/2
  Product2/1 -> Add1/1
  Divide/1 -> Mux/3
  Sqrt/1 -> Divide/2, Mux/1
  Add/1 -> Divide/1
  Product1/1 -> Add/2
  Product/1 -> Add/1
  Ydot/1 -> Product1/2, Product2/2
  Xdot/1 -> Product/2, Product3/2
  Y/1 -> Math Function1/1, Product1/1, Product3/1, Trigonometric Function/1
  X/1 -> Math Function/1, Product/1, Product2/1, Trigonometric Function/2
  Trigonometric Function/1 -> Mux/2
  Sum/1 -> Sqrt/1, Divide1/2
  Math Function/1 -> Sum/1
  Math Function1/1 -> Sum/2

== system Contact_Forces_Lib/2D/Circle to Finite Line Force/Forces/Resolve Forces/Friction/VCirPt ==
  wz : Inport
  X sep : Inport  Port=2
  Constant : Constant  Value=line_depth
  Product : Product
  Product1 : Product
  Sign1 : Signum
  Subtract : Sum  Inputs=+-
  vCir : Outport
  wires:
  wz/1 -> Product1/1
  Product1/1 -> vCir/1
  Product/1 -> Subtract/2
  Sign1/1 -> Product/1
  X sep/1 -> Subtract/1, Sign1/1
  Constant/1 -> Product/2
  Subtract/1 -> Product1/2

== system Contact_Forces_Lib/2D/Circle to Finite Line Force Enabled/Forces/Resolve Forces/Friction/VCirPt ==
  wz : Inport
  X sep : Inport  Port=2
  Constant : Constant  Value=line_depth
  Product : Product
  Product1 : Product
  Sign1 : Signum
  Subtract : Sum  Inputs=+-
  vCir : Outport
  wires:
  Subtract/1 -> Product1/2
  Constant/1 -> Product/2
  X sep/1 -> Sign1/1, Subtract/1
  Sign1/1 -> Product/1
  Product/1 -> Subtract/2
  Product1/1 -> vCir/1
  wz/1 -> Product1/1

== system Contact_Forces_Lib/2D/Circle to Ring Force/Forces/Ff/Resolve Ff/Ff in CirB ==
  Ff : Inport
  azm : Inport  Port=2
  Divide1 : Product  Inputs=**
  Divide2 : Product  Inputs=**
  Gain1 : Gain
  Gain3 : Gain  Gain=-1
  cos : Trigonometry
  deg2rad : Gain  Gain=pi/180
  sin : Trigonometry  Operator=cos
  FxRinB : Outport
  FyRinB : Outport  Port=2
  wires:
  Gain1/1 -> Divide2/1, Divide1/1
  azm/1 -> deg2rad/1
  Divide2/1 -> FyRinB/1
  cos/1 -> Gain3/1
  sin/1 -> Divide2/2
  deg2rad/1 -> sin/1, cos/1
  Divide1/1 -> FxRinB/1
  Ff/1 -> Gain1/1
  Gain3/1 -> Divide1/2
